simulink model "Simulink_ControllerTF_BlaneRev"  (R2020b)
settings: Solver=VariableStepAuto  StartTime=0.0  StopTime=3200  RelTol=1e-3
values from neighbouring files (symbols this model uses):
  A = [a2, a1, a0]    [Controller_ARMAX_BlaneRev.m]    (also in Controller_SS_BlaneRev.m; Controller_TF_BlaneRev.m = [a1, a0])
  B = [b2, b1, b0]    [Controller_ARMAX_BlaneRev.m]    (also in Controller_SS_BlaneRev.m; Controller_TF_BlaneRev.m = [b1, b0])
  b = double(sol.b)    [Controller_ARMAX_BlaneRev.m]    (also in Controller_SS_BlaneRev.m; Controller_TF_BlaneRev.m = double(sol))
  b_tun = 1    [Controller_ARMAX_BlaneRev.m]    (also in Controller_SS_BlaneRev.m = 0.04062; Controller_TF_BlaneRev.m = 0.008893)
  Gp = tf(sysARMAX)    [Controller_ARMAX_BlaneRev.m]    (also in Controller_SS_BlaneRev.m = tf(B, A, Ts2); Controller_TF_BlaneRev.m = tf(sysTF))
  Gp_cont = d2c(Gp_origin, 'zoh')    [Controller_ARMAX_BlaneRev.m]    (also in Controller_SS_BlaneRev.m; Controller_TF_BlaneRev.m = d2c(Gp, 'zoh'))
  I = double(sol.I)    [Controller_ARMAX_BlaneRev.m]    (also in Controller_SS_BlaneRev.m; Controller_TF_BlaneRev.m)
  I_tun = .06907    (= 0.06907)    [Controller_ARMAX_BlaneRev.m]    (also in Controller_SS_BlaneRev.m = 0.1006; Controller_TF_BlaneRev.m = 0.08704)
  P = double(sol.P)    [Controller_ARMAX_BlaneRev.m]    (also in Controller_SS_BlaneRev.m; Controller_TF_BlaneRev.m)
  P_tun = 5.628    [Controller_ARMAX_BlaneRev.m]    (also in Controller_SS_BlaneRev.m = 7.185; Controller_TF_BlaneRev.m = 3.173)
  Ts = .4    (= 0.4)    [Controller_ARMAX_BlaneRev.m]    (also in Controller_SS_BlaneRev.m; Controller_TF_BlaneRev.m; systemIdentification_47414_Blane.m = 0.2; systemIdentification_48404_Blane.m = 1)
  Ts3 = 1    [Controller_ARMAX_BlaneRev.m]    (also in Controller_SS_BlaneRev.m; Controller_TF_BlaneRev.m)
undefined symbols (not defined in the file or in its folder): DiscIntNeverNeededParam, K_ant
libraries: simulink_extras x7
settings Model: Creator=Blane Brinkley  LastModifiedBy=Blane Brinkley

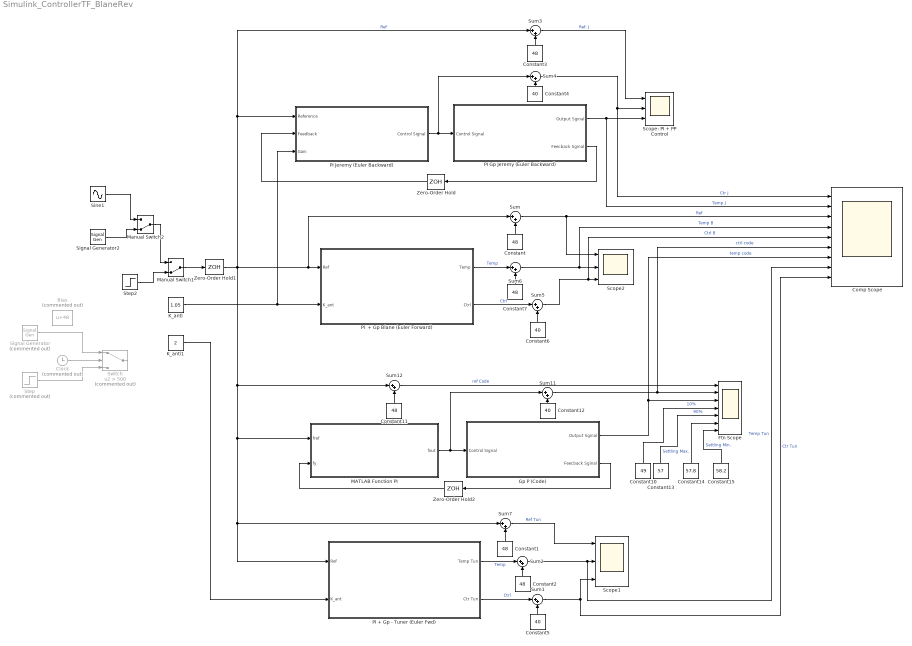
== system Simulink_ControllerTF_BlaneRev ==
  Bias : Bias  Commented=on  Bias=48
  Clock : Clock  Commented=on
  Comp Scope : Scope  NumInputPorts=9
  Constant{,1..3,7,11} (6 alike) : Constant  Value=48
  Constant10 : Constant  Value=49
  Constant{4..6,12} (4 alike) : Constant  Value=40
  Constant13 : Constant  Value=57
  Constant14 : Constant  Value=57.8
  Constant15 : Constant  Value=58.2
  Ftn Scope : Scope  NumInputPorts=7
  Gp P (Code) : Subsystem
  K_anti : Constant  Value=1.05
  K_anti1 : Constant  Value=2
  MATLAB Function PI : MATLAB Function  TreatAsAtomicUnit=on
  Manual Switch1 : ManualSwitch  CurrentSetting=0
  Manual Switch2 : ManualSwitch  CurrentSetting=0
  PI  + Gp Blane (Euler Forward) : Subsystem
  "PI + Gp - Tuner (Euler Fwd)  " : Subsystem
  PI Gp Jeremy (Euler Backward) : Subsystem
  PI Jeremy (Euler Backward) : Subsystem
  Scope1 : Scope  NumInputPorts=3
  Scope2 : Scope  NumInputPorts=3
  Scope: PI + PP Control : Scope  NumInputPorts=3
  Signal Generator : SignalGenerator  Commented=on  WaveForm=square  Amplitude=10  Frequency=1/200
  Signal Generator2 : SignalGenerator  WaveForm=square  Amplitude=5  Frequency=1/1600
  Sine1 : Sin  Amplitude=10  Frequency=1/1200*6.28  SampleTime=0
  Step : Step  Commented=on  Time=100  Before=-21  After=0  SampleTime=Ts
  Step2 : Step  Time=0  After=10  SampleTime=Ts
  Sum{,1..7,11..12} (10 alike) : Sum  Inputs=|++
  Switch : Switch  Commented=on  Criteria=u2 > Threshold  Threshold=500
  Zero-Order Hold : ZeroOrderHold  SampleTime=Ts3
  Zero-Order Hold1 : ZeroOrderHold  SampleTime=Ts3
  Zero-Order Hold2 : ZeroOrderHold  SampleTime=Ts3
  wires:
  K_anti/1 -> PI  + Gp Blane (Euler Forward)/2(K_ant), PI Jeremy (Euler Backward)/3(Gain)
  PI  + Gp Blane (Euler Forward)/1(Temp) -> Sum6/1  "Temp"
  Constant/1 -> Sum/2
  PI  + Gp Blane (Euler Forward)/2(Ctrl) -> Sum5/1  "Ctrl"
  Sum5/1 -> Comp Scope/5, Scope2/3  "Ctrl B"
  Signal Generator/1 -> Switch/1
  Step/1 -> Switch/3
  Constant7/1 -> Sum6/2
  Constant6/1 -> Sum5/2
  Sum6/1 -> Comp Scope/4, Scope2/2  "Temp B"
  Clock/1 -> Switch/2
  Sum/1 -> Scope2/1, Comp Scope/3  "Ref"
  PI Jeremy (Euler Backward)/1(Control Signal) -> Sum4/1, PI Gp Jeremy (Euler Backward)/1(Control Signal)
  Sum4/1 -> Comp Scope/1, Scope: PI + PP Control/2  "Ctr J"
  PI Gp Jeremy (Euler Backward)/1(Output Sginal) -> Comp Scope/2, Scope: PI + PP Control/3  "Temp J"
  Manual Switch1/1 -> Zero-Order Hold1/1
  Constant4/1 -> Sum4/2
  Constant3/1 -> Sum3/2
  Sum3/1 -> Scope: PI + PP Control/1  "Ref. J"
  PI Gp Jeremy (Euler Backward)/2(Feecback Sginal) -> Zero-Order Hold/1
  Zero-Order Hold/1 -> PI Jeremy (Euler Backward)/2(Feedback)
  Constant11/1 -> Sum12/2
  Gp P (Code)/2(Feecback Sginal) -> Zero-Order Hold2/1
  Constant12/1 -> Sum11/2
  MATLAB Function PI/1(fout) -> Sum11/1, Gp P (Code)/1(Control Signal)
  Sum11/1 -> Ftn Scope/2, Comp Scope/6  "ctrl code"
  Sum12/1 -> Ftn Scope/1  "ref Code"
  Gp P (Code)/1(Output Sginal) -> Ftn Scope/3, Comp Scope/7  "temp code"
  Zero-Order Hold2/1 -> MATLAB Function PI/2(fy)
  Zero-Order Hold1/1 -> Sum/1, PI  + Gp Blane (Euler Forward)/1(Ref), Sum7/1, "PI + Gp - Tuner (Euler Fwd)  "/1(Ref), MATLAB Function PI/1(fref), Sum12/1, PI Jeremy (Euler Backward)/1(Reference), Sum3/1  "Ref"
  Sum1/1 -> Scope1/3, Comp Scope/9  "Ctr Tun"
  Constant1/1 -> Sum7/2
  "PI + Gp - Tuner (Euler Fwd)  "/1(Temp Tun) -> Sum2/1  "Temp"
  "PI + Gp - Tuner (Euler Fwd)  "/2(Ctr Tun) -> Sum1/1  "Ctrl"
  Constant2/1 -> Sum2/2
  Sum2/1 -> Scope1/2, Comp Scope/8  "Temp Tun"
  Constant5/1 -> Sum1/2
  Sum7/1 -> Scope1/1  "Ref Tun"
  K_anti1/1 -> "PI + Gp - Tuner (Euler Fwd)  "/2(K_ant)
  Step2/1 -> Manual Switch1/2
  Sine1/1 -> Manual Switch2/1
  Signal Generator2/1 -> Manual Switch2/2
  Manual Switch2/1 -> Manual Switch1/1
  Constant10/1 -> Ftn Scope/4  "10%"
  Constant13/1 -> Ftn Scope/5  "90%"
  Constant14/1 -> Ftn Scope/6  "Settling Max."
  Constant15/1 -> Ftn Scope/7  "Settling Min."

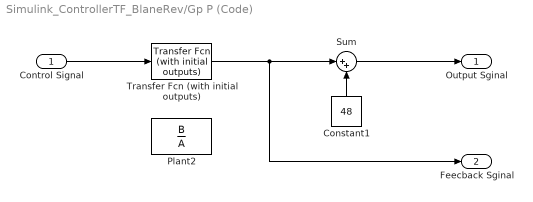
== system Simulink_ControllerTF_BlaneRev/Gp P (Code) ==
  Control Signal : Inport
  Constant1 : Constant  Value=48
  Plant2 : DiscreteTransferFcn  Numerator=B  Denominator=A  SampleTime=0.4
  Sum : Sum  Inputs=|++
  Transfer Fcn (with initial outputs) : simulink_extras/Additional Linear/Transfer Fcn (with initial outputs)  N=Gp_cont.Numerator{1}  D=Gp_cont.Denominator{1}  Y0=0  U0=0
  Output Sginal : Outport
  Feecback Sginal : Outport  Port=2
  wires:
  Transfer Fcn (with initial outputs)/1 -> Feecback Sginal/1, Sum/1
  Sum/1 -> Output Sginal/1
  Constant1/1 -> Sum/2
  Control Signal/1 -> Transfer Fcn (with initial outputs)/1

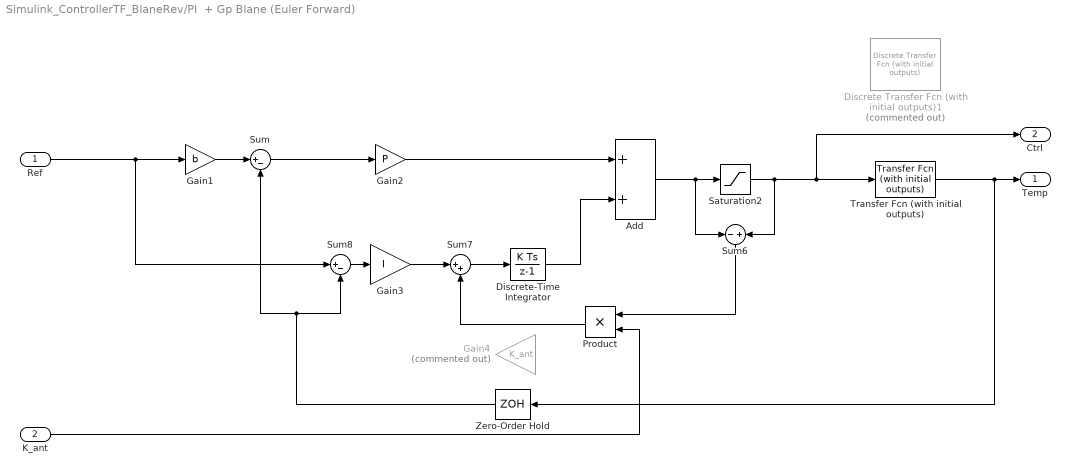
== system Simulink_ControllerTF_BlaneRev/PI  + Gp Blane (Euler Forward) ==
  Ref : Inport
  K_ant : Inport  Port=2
  Add : Sum
  Discrete Transfer Fcn (with initial outputs)1 : simulink_extras/Additional Discrete/Discrete Transfer Fcn (with initial outputs)  Commented=on  N=Gp.Numerator{1}  D=Gp.Denominator{1}  U0=[1]  Y0=0  TS=Ts
      settings: SourceProductBaseCode=SL
  Discrete-Time Integrator : DiscreteIntegrator  SampleTime=Ts3  ICPrevOutput=DiscIntNeverNeededParam  ICPrevScaledInput=DiscIntNeverNeededParam
  Gain1 : Gain  Gain=b
  Gain2 : Gain  Gain=P
  Gain3 : Gain  Gain=I
  Gain4 : Gain  Commented=on  Gain=K_ant
  Product : Product
  Saturation2 : Saturate  UpperLimit=60  LowerLimit=-40
  Sum : Sum  Inputs=|+-
  Sum6 : Sum  Inputs=-+
  Sum7 : Sum  Inputs=|++
  Sum8 : Sum  Inputs=|+-
  Transfer Fcn (with initial outputs) : simulink_extras/Additional Linear/Transfer Fcn (with initial outputs)  N=Gp_cont.Numerator{1}  D=Gp_cont.Denominator{1}  Y0=0  U0=0
  Zero-Order Hold : ZeroOrderHold  SampleTime=Ts3
  Temp : Outport
  Ctrl : Outport  Port=2
  wires:
  Gain1/1 -> Sum/1
  Sum/1 -> Gain2/1
  Sum8/1 -> Gain3/1
  Sum6/1 -> Product/1
  Add/1 -> Sum6/1, Saturation2/1
  Sum7/1 -> Discrete-Time Integrator/1
  Transfer Fcn (with initial outputs)/1 -> Zero-Order Hold/1, Temp/1
  Gain2/1 -> Add/1
  Product/1 -> Sum7/2
  Discrete-Time Integrator/1 -> Add/2
  Gain3/1 -> Sum7/1
  Saturation2/1 -> Sum6/2, Transfer Fcn (with initial outputs)/1, Ctrl/1
  Zero-Order Hold/1 -> Sum8/2, Sum/2
  Ref/1 -> Sum8/1, Gain1/1
  K_ant/1 -> Product/2

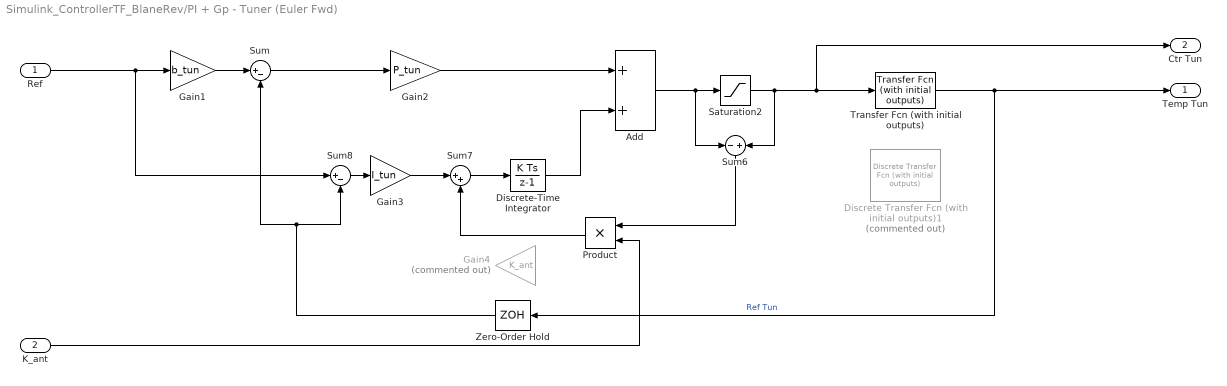
== system Simulink_ControllerTF_BlaneRev/PI + Gp - Tuner (Euler Fwd)   ==
  Ref : Inport
  K_ant : Inport  Port=2
  Add : Sum
  Discrete Transfer Fcn (with initial outputs)1 : simulink_extras/Additional Discrete/Discrete Transfer Fcn (with initial outputs)  Commented=on  N=Gp.Numerator{1}  D=Gp.Denominator{1}  U0=[1]  Y0=0  TS=Ts
      settings: SourceProductBaseCode=SL
  Discrete-Time Integrator : DiscreteIntegrator  SampleTime=Ts3  ICPrevOutput=DiscIntNeverNeededParam  ICPrevScaledInput=DiscIntNeverNeededParam
  Gain1 : Gain  Gain=b_tun
  Gain2 : Gain  Gain=P_tun
  Gain3 : Gain  Gain=I_tun
  Gain4 : Gain  Commented=on  Gain=K_ant
  Product : Product
  Saturation2 : Saturate  UpperLimit=60  LowerLimit=-40
  Sum : Sum  Inputs=|+-
  Sum6 : Sum  Inputs=-+
  Sum7 : Sum  Inputs=|++
  Sum8 : Sum  Inputs=|+-
  Transfer Fcn (with initial outputs) : simulink_extras/Additional Linear/Transfer Fcn (with initial outputs)  N=Gp_cont.Numerator{1}  D=Gp_cont.Denominator{1}  Y0=0  U0=0
  Zero-Order Hold : ZeroOrderHold  SampleTime=Ts3
  Temp Tun : Outport
  Ctr Tun : Outport  Port=2
  wires:
  Gain1/1 -> Sum/1
  Sum/1 -> Gain2/1
  Sum8/1 -> Gain3/1
  Sum6/1 -> Product/1
  Add/1 -> Sum6/1, Saturation2/1
  Sum7/1 -> Discrete-Time Integrator/1
  Gain2/1 -> Add/1
  Product/1 -> Sum7/2
  Discrete-Time Integrator/1 -> Add/2
  Gain3/1 -> Sum7/1
  Saturation2/1 -> Sum6/2, Transfer Fcn (with initial outputs)/1, Ctr Tun/1
  Zero-Order Hold/1 -> Sum8/2, Sum/2
  Ref/1 -> Sum8/1, Gain1/1
  K_ant/1 -> Product/2
  Transfer Fcn (with initial outputs)/1 -> Temp Tun/1, Zero-Order Hold/1  "Ref Tun"

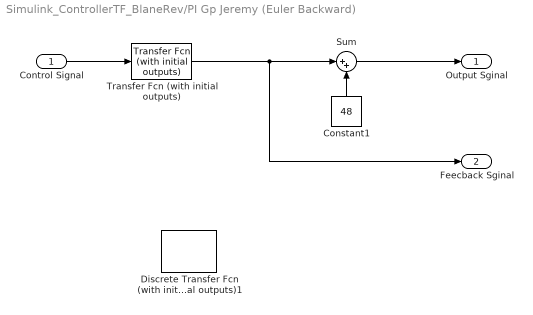
== system Simulink_ControllerTF_BlaneRev/PI Gp Jeremy (Euler Backward) ==
  Control Signal : Inport
  Constant1 : Constant  Value=48
  Discrete Transfer Fcn (with initial outputs)1 : simulink_extras/Additional Discrete/Discrete Transfer Fcn (with initial outputs)  N=Gp.Numerator{1}  D=Gp.Denominator{1}  U0=[1]  Y0=0  TS=Ts
      settings: SourceProductBaseCode=SL
  Sum : Sum  Inputs=|++
  Transfer Fcn (with initial outputs) : simulink_extras/Additional Linear/Transfer Fcn (with initial outputs)  N=Gp_cont.Numerator{1}  D=Gp_cont.Denominator{1}  Y0=0  U0=0
  Output Sginal : Outport
  Feecback Sginal : Outport  Port=2
  wires:
  Transfer Fcn (with initial outputs)/1 -> Feecback Sginal/1, Sum/1
  Sum/1 -> Output Sginal/1
  Constant1/1 -> Sum/2
  Control Signal/1 -> Transfer Fcn (with initial outputs)/1

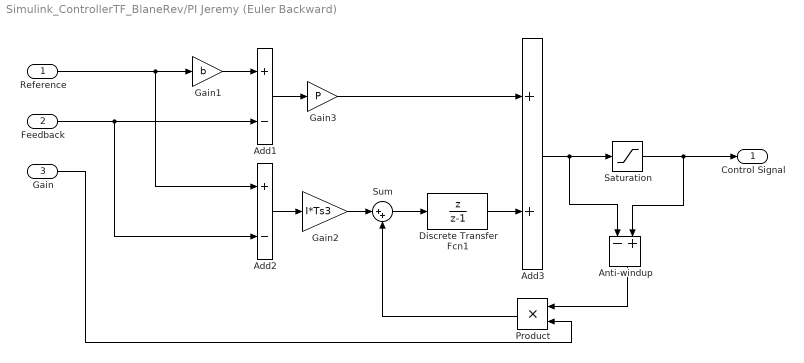
== system Simulink_ControllerTF_BlaneRev/PI Jeremy (Euler Backward) ==
  Reference : Inport
  Feedback : Inport  Port=2
  Gain : Inport  Port=3
  Add1 : Sum  Inputs=+-
  Add2 : Sum  Inputs=+-
  Add3 : Sum
  Anti-windup : Sum  Inputs=-+
  Discrete Transfer Fcn1 : DiscreteTransferFcn  Numerator=[1 0]  Denominator=[1 -1]  SampleTime=Ts3
  Gain1 : Gain  Gain=b
  Gain2 : Gain  Gain=I*Ts3
  Gain3 : Gain  Gain=P
  Product : Product
  Saturation : Saturate  UpperLimit=60  LowerLimit=-40
  Sum : Sum  Inputs=|++
  Control Signal : Outport
  wires:
  Gain1/1 -> Add1/1
  Feedback/1 -> Add1/2, Add2/2
  Reference/1 -> Add2/1, Gain1/1
  Sum/1 -> Discrete Transfer Fcn1/1
  Discrete Transfer Fcn1/1 -> Add3/2
  Saturation/1 -> Anti-windup/2, Control Signal/1
  Product/1 -> Sum/2
  Add3/1 -> Anti-windup/1, Saturation/1
  Add1/1 -> Gain3/1
  Gain3/1 -> Add3/1
  Add2/1 -> Gain2/1
  Gain2/1 -> Sum/1
  Anti-windup/1 -> Product/1
  Gain/1 -> Product/2

== matlab function Simulink_ControllerTF_BlaneRev/MATLAB Function PI ==
  data: fref input; fout output; fy input
function fout = fcn(fref, fy)
%%%%%%%%%%%%%%%%%%%%%%%%%%%%%%%%%%%%%%%%%%%%%%%%%%%%%%%
% PID + LP + PP for ARMAX
% Input : fref - reference signal
%         fy   - feedback signal
% Output: fout - control signal
%%%%%%%%%%%%%%%%%%%%%%%%%%%%%%%%%%%%%%%%%%%%%%%%%%%%%%%
% Variable Initialisation
persistent  fI_prev fIA_prev fant;

% Blane - SLOW (61.47 sec):
Ts = 1;        
P = 9.4233;     
I = .1209;    
b = .7155;    
Kant = 1; 

% % Blane - FAST (61.47 sec):
% Ts = 1;        
% P = 49.9724;     
% I = 1.9620;    
% b = .3351;    
% Kant = 1; 

% Jeremy (107.45 sec)
% Ts = 1;        
% P = 3.173;     
% I = 0.08704;    
% b = 0.008893;  
% Kant = 2;

if isempty(fI_prev)
    fI_prev = 0;
    fIA_prev = 0;
    fant = 0;
    
end

fErr = fref - fy;

% P
fP = P*(b*fref - fy);
% I
fI = fI_prev + fErr*I*Ts;
% Kant = 10
fIA = fIA_prev + Kant*fant;

fsum = fP + fI + fIA;

if fsum > 60
    fout = 60;
elseif fsum < (-40)
    fout = -40;
else
    fout = fsum;
end

% Update values
fI_prev = fI;
fIA_prev = fIA;
fant = fout - fsum;
end
